simulink model "schemaclasica_regualtorPI"  (R2017b)
settings: Solver=VariableStepAuto  StartTime=0.0  StopTime=1000  RelTol=1e-3
values from neighbouring files (symbols this model uses):
  k = 0.035    [modelare.m]
  k1 = 0.624    [modelare.m]
  k2 = -0.015    [modelare.m]
  k3 = -0.0006    [modelare.m]
libraries: simulink x1
settings Model: Creator=alinvoicu26  LastModifiedBy=alinvoicu26

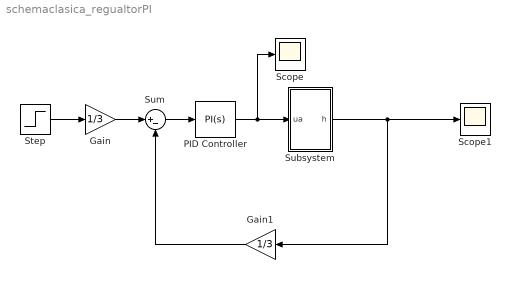
== system schemaclasica_regualtorPI ==
  Gain : Gain  Gain=1/3
  Gain1 : Gain  Gain=1/3
  PID Controller : simulink/Continuous/PID Controller  Controller=PI  TimeDomain=Continuous-time  SampleTime=-1  IntegratorMethod=Forward Euler  FilterMethod=Forward Euler  Form=Parallel  UseFilter=on  ControllerParametersSource=internal  P=2.395  I=2.395/160  D=0  N=100  InitialConditionSource=internal  InitialConditionForIntegrator=5  InitialConditionForFilter=0  ExternalReset=none  LimitOutput=off  UpperSaturationLimit=inf  LowerSaturationLimit=-inf  LinearizeAsGain=on  AntiWindupMode=none  Kb=1  TrackingMode=off  Kt=1  PParamMin=[]  PParamMax=[]  IParamMin=[]  IParamMax=[]  DParamMin=[]  DParamMax=[]  NParamMin=[]  NParamMax=[]  KbParamMin=[]  KbParamMax=[]  KtParamMin=[]  KtParamMax=[]  POutMin=[]  POutMax=[]  IOutMin=[]  IOutMax=[]  DOutMin=[]  DOutMax=[]  NOutMin=[]  NOutMax=[]  KbOutMin=[]  KbOutMax=[]  KtOutMin=[]  KtOutMax=[]  IntegratorOutMin=[]  IntegratorOutMax=[]  FilterOutMin=[]  FilterOutMax=[]  SumOutMin=[]  SumOutMax=[]  SumI1OutMin=[]  SumI1OutMax=[]  SumI2OutMin=[]  SumI2OutMax=[]  SumI3OutMin=[]  SumI3OutMax=[]  SumDOutMin=[]  SumDOutMax=[]  SaturationOutMin=[]  SaturationOutMax=[]  IntegratorContinuousStateAttributes=''  IntegratorStateMustResolveToSignalObject=off  IntegratorRTWStateStorageClass=Auto  FilterContinuousStateAttributes=''  FilterStateMustResolveToSignalObject=off  FilterRTWStateStorageClass=Auto  DifferentiatorICPrevScaledInput=0  DifferentiatorOutMin=[]  DifferentiatorOutMax=[]  InitialConditionSetting=State (most efficient)  FilterDiffOutCoefMin=[]  FilterDiffOutCoefMax=[]  SumDenOutMin=[]  SumDenOutMax=[]  SumNumOutMin=[]  SumNumOutMax=[]  ReciprocalOutMin=[]  ReciprocalOutMax=[]  DivideOutMin=[]  DivideOutMax=[]  TunerSelectOption=Transfer Function Based (PID Tuner App)
  Scope : Scope
  Scope1 : Scope
  Step : Step  Before=10.5  After=13  SampleTime=0
  Subsystem : Subsystem
  Sum : Sum  Inputs=|+-
  wires:
  Step/1 -> Gain/1
  Gain/1 -> Sum/1
  Sum/1 -> PID Controller/1
  Gain1/1 -> Sum/2
  Subsystem/1("h ") -> Scope1/1, Gain1/1
  PID Controller/1 -> Scope/1, Subsystem/1(ua)

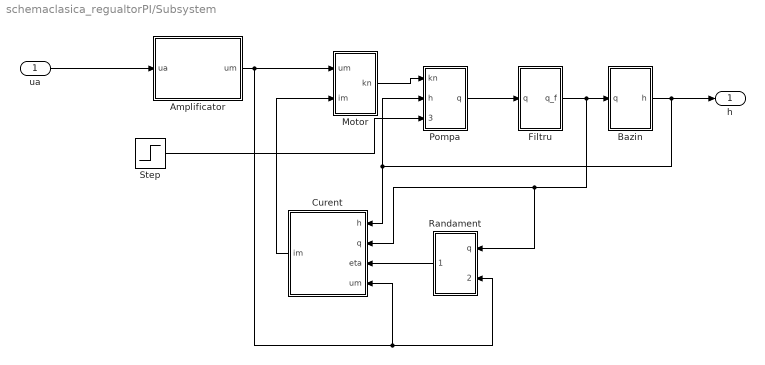
== system schemaclasica_regualtorPI/Subsystem ==
  ua : Inport
  Amplificator : Subsystem
  "Bazin " : Subsystem
  Curent : Subsystem
  "Filtru " : Subsystem
  Motor : Subsystem
  "Pompa " : Subsystem
  Randament : Subsystem
  Step : Step  Time=300  After=0.01  SampleTime=0
  "h " : Outport
  wires:
  Amplificator/1("um ") -> Motor/1(um), Curent/4(um), Randament/2(um)
  Motor/1(kn) -> "Pompa "/1(kn)
  "Filtru "/1("q_f ") -> Randament/1(q), Curent/2(q), "Bazin "/1(q)
  "Bazin "/1("h ") -> Curent/1("h "), "Pompa "/2(h), "h "/1
  "Pompa "/1("q ") -> "Filtru "/1("q ")
  Randament/1("eta ") -> Curent/3(eta)
  Curent/1("im ") -> Motor/2("im ")
  ua/1 -> Amplificator/1("ua ")
  Step/1 -> "Pompa "/3(perturabtie k)

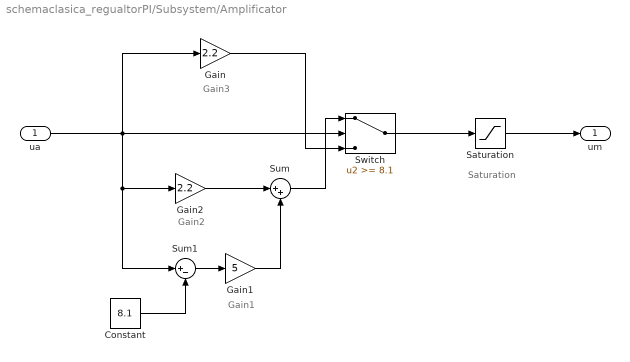
== system schemaclasica_regualtorPI/Subsystem/Amplificator ==
  note: Saturation
  note: Gain3
  note: Gain2
  note: Gain1
  "ua " : Inport
  Constant : Constant  Value=8.1
  Gain : Gain  Gain=2.2
  Gain1 : Gain  Gain=5
  Gain2 : Gain  Gain=2.2
  Saturation : Saturate  UpperLimit=22  LowerLimit=0
  Sum : Sum  Inputs=|++
  Sum1 : Sum  Inputs=|+-
  Switch : Switch  Threshold=8.1
  "um " : Outport
  wires:
  Switch/1 -> Saturation/1
  Gain2/1 -> Sum/1
  Sum/1 -> Switch/1
  "ua "/1 -> Sum1/1, Gain2/1, Gain/1, Switch/2
  Gain/1 -> Switch/3
  Gain1/1 -> Sum/2
  Sum1/1 -> Gain1/1
  Constant/1 -> Sum1/2
  Saturation/1 -> "um "/1

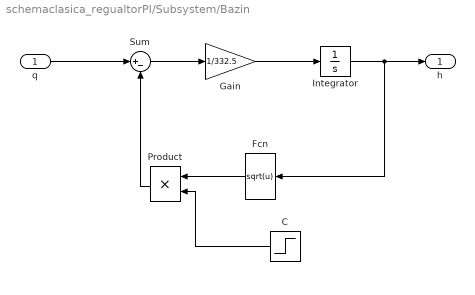
== system schemaclasica_regualtorPI/Subsystem/Bazin  ==
  q : Inport
  C : Step  Time=250  Before=9  After=9  SampleTime=0
  Fcn : Fcn  Expr=sqrt(u)
  Gain : Gain  Gain=1/332.5
  Integrator : Integrator  InitialCondition=10.5
  Product : Product
  Sum : Sum  Inputs=|+-
  "h " : Outport
  wires:
  q/1 -> Sum/1
  Integrator/1 -> Fcn/1, "h "/1
  Gain/1 -> Integrator/1
  Sum/1 -> Gain/1
  Fcn/1 -> Product/1
  Product/1 -> Sum/2
  C/1 -> Product/2

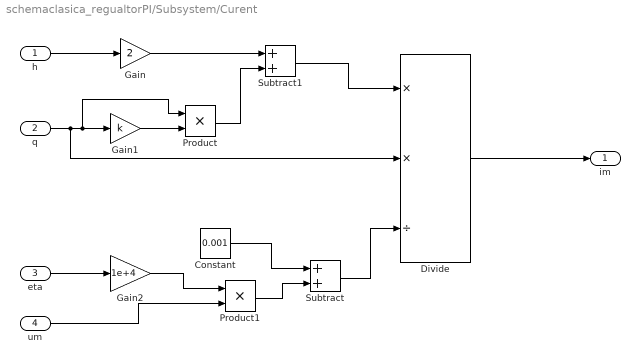
== system schemaclasica_regualtorPI/Subsystem/Curent ==
  "h " : Inport
  q : Inport  Port=2
  eta : Inport  Port=3
  um : Inport  Port=4
  Constant : Constant  Value=0.001
  Divide : Product  Inputs=**/
  Gain : Gain  Gain=2
  Gain1 : Gain  Gain=k
  Gain2 : Gain  Gain=1e+4
  Product : Product
  Product1 : Product
  Subtract : Sum
  Subtract1 : Sum
  "im " : Outport
  wires:
  Constant/1 -> Subtract/1
  Gain/1 -> Subtract1/1
  q/1 -> Divide/2, Product/1, Gain1/1
  Divide/1 -> "im "/1
  Subtract1/1 -> Divide/1
  Gain2/1 -> Product1/1
  "h "/1 -> Gain/1
  Product1/1 -> Subtract/2
  Subtract/1 -> Divide/3
  eta/1 -> Gain2/1
  Product/1 -> Subtract1/2
  um/1 -> Product1/2
  Gain1/1 -> Product/2

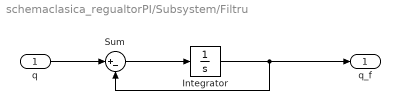
== system schemaclasica_regualtorPI/Subsystem/Filtru  ==
  "q " : Inport
  Integrator : Integrator  InitialCondition=29.2
  Sum : Sum  Inputs=|+-
  "q_f " : Outport
  wires:
  Sum/1 -> Integrator/1
  "q "/1 -> Sum/1
  Integrator/1 -> "q_f "/1, Sum/2

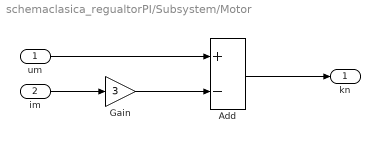
== system schemaclasica_regualtorPI/Subsystem/Motor ==
  um : Inport
  "im " : Inport  Port=2
  Add : Sum  Inputs=+-
  Gain : Gain  Gain=3
  kn : Outport
  wires:
  "im "/1 -> Gain/1
  Add/1 -> kn/1
  Gain/1 -> Add/2
  um/1 -> Add/1

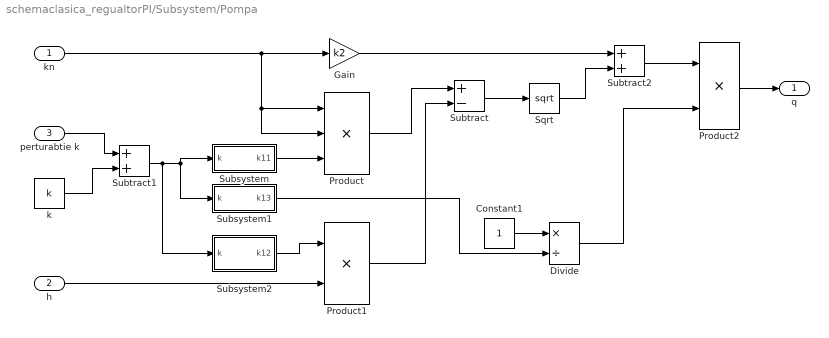
== system schemaclasica_regualtorPI/Subsystem/Pompa  ==
  kn : Inport
  h : Inport  Port=2
  perturabtie k : Inport  Port=3
  Constant1 : Constant
  Divide : Product  Inputs=*/
  Gain : Gain  Gain=k2
  Product : Product  Inputs=3
  Product1 : Product
  Product2 : Product
  Sqrt : Sqrt  SaturateOnIntegerOverflow=on
  Subsystem : Subsystem
  Subsystem1 : Subsystem
  Subsystem2 : Subsystem
  Subtract : Sum  Inputs=+-
  Subtract1 : Sum
  Subtract2 : Sum
  k : Constant  Value=k
  "q " : Outport
  wires:
  kn/1 -> Product/2, Product/1, Gain/1
  k/1 -> Subtract1/2
  perturabtie k/1 -> Subtract1/1
  Subsystem/1(k11) -> Product/3
  Subtract1/1 -> Subsystem2/1(k), Subsystem1/1(k), Subsystem/1(k)
  Subsystem2/1(k12) -> Product1/1
  h/1 -> Product1/2
  Subsystem1/1(k13) -> Divide/2
  Constant1/1 -> Divide/1
  Product/1 -> Subtract/1
  Product1/1 -> Subtract/2
  Subtract/1 -> Sqrt/1
  Gain/1 -> Subtract2/1
  Sqrt/1 -> Subtract2/2
  Subtract2/1 -> Product2/1
  Divide/1 -> Product2/2
  Product2/1 -> "q "/1

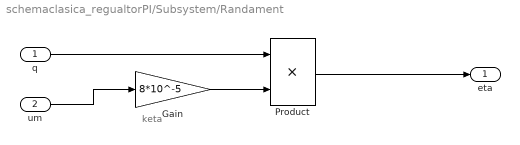
== system schemaclasica_regualtorPI/Subsystem/Randament ==
  note: keta
  q : Inport
  um : Inport  Port=2
  Gain : Gain  Gain=8*10^-5
  Product : Product
  "eta " : Outport
  wires:
  Gain/1 -> Product/2
  q/1 -> Product/1
  um/1 -> Gain/1
  Product/1 -> "eta "/1

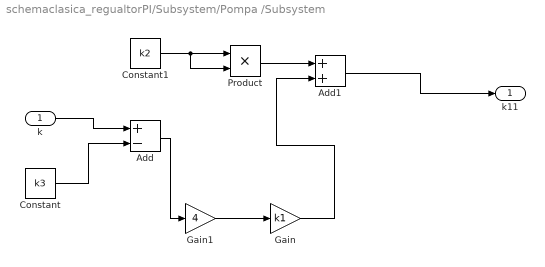
== system schemaclasica_regualtorPI/Subsystem/Pompa /Subsystem ==
  k : Inport
  Add : Sum  Inputs=+-
  Add1 : Sum
  Constant : Constant  Value=k3
  Constant1 : Constant  Value=k2
  Gain : Gain  Gain=k1
  Gain1 : Gain  Gain=4
  Product : Product
  k11 : Outport
  wires:
  k/1 -> Add/1
  Constant/1 -> Add/2
  Constant1/1 -> Product/2, Product/1
  Product/1 -> Add1/1
  Add1/1 -> k11/1
  Gain/1 -> Add1/2
  Gain1/1 -> Gain/1
  Add/1 -> Gain1/1

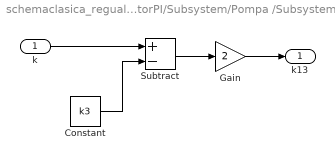
== system schemaclasica_regualtorPI/Subsystem/Pompa /Subsystem1 ==
  k : Inport
  Constant : Constant  Value=k3
  Gain : Gain  Gain=2
  Subtract : Sum  Inputs=+-
  k13 : Outport
  wires:
  Constant/1 -> Subtract/2
  k/1 -> Subtract/1
  Subtract/1 -> Gain/1
  Gain/1 -> k13/1

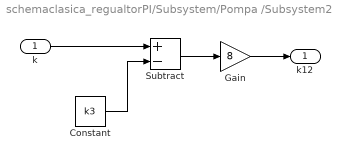
== system schemaclasica_regualtorPI/Subsystem/Pompa /Subsystem2 ==
  k : Inport
  Constant : Constant  Value=k3
  Gain : Gain  Gain=8
  Subtract : Sum  Inputs=+-
  k12 : Outport
  wires:
  k/1 -> Subtract/1
  Gain/1 -> k12/1
  Subtract/1 -> Gain/1
  Constant/1 -> Subtract/2
